simulink model "waterTank"  (Simulink 8.3)
settings: Solver=ode45  StartTime=0.0  StopTime=16  RelTol=1e-3
settings Model: Creator=yangg  LastModifiedBy=yangg
settings DataIOCC: MaxDataPoints=1000000  SaveFormat=StructureWithTime  SignalLoggingSaveFormat=Dataset
settings DebuggingCC: UnderspecifiedInitializationDetection=Simplified  StateNameClashWarn=none
settings GRTTargetCC: CombineOutputUpdateFcns=on  GRTInterface=off

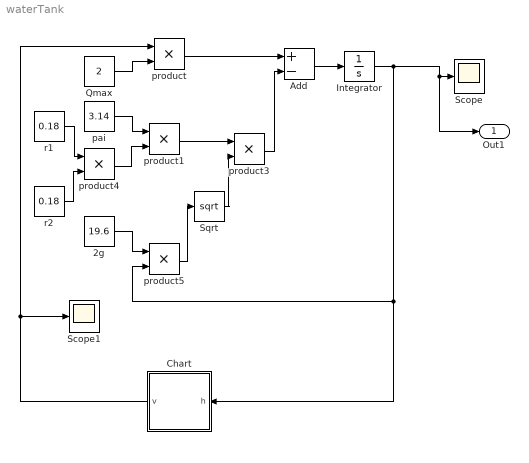
== system waterTank ==
  2g : Constant  Value=19.6
  Add : Sum  Inputs=+-  SampleTime=0.001
  Chart : Stateflow chart  TreatAsAtomicUnit=on
  Integrator : Integrator  InitialCondition=4.5
  Qmax : Constant  Value=2
  Scope : Scope
      settings: TimeRange=6.400000000000001  YMin=3  YMax=6.5  MaxDataPoints=50000000
  Scope1 : Scope
  Sqrt : Sqrt  SampleTime=0.001  SaturateOnIntegerOverflow=on
  pai : Constant  Value=3.14
  product{,1,3..5} (5 alike) : Product  Inputs=**  SampleTime=0.001
  r1 : Constant  Value=0.18
  r2 : Constant  Value=0.18
  Out1 : Outport
  wires:
  Qmax/1 -> product/2
  pai/1 -> product1/1
  product4/1 -> product1/2
  r1/1 -> product4/1
  r2/1 -> product4/2
  2g/1 -> product5/1
  product1/1 -> product3/1
  product/1 -> Add/1
  product3/1 -> Add/2
  Add/1 -> Integrator/1
  Integrator/1 -> Out1/1, Scope/1, Chart/1(h), product5/2
  product5/1 -> Sqrt/1
  Sqrt/1 -> product3/2
  Chart/1(v) -> Scope1/1, product/1

== stateflow chart Chart ==
  settings: updateMethod=DISCRETE  sampleTime=1
  state on
    entry:v=1;
  state off
    entry:v=0;
  (default) -> on
  on -> off : [h>=5.9]
  off -> on : [h<=4.1]
  data: h input double; v output double
